simulink model "FDM_Degradation_nmmap"  (R2020b)
settings: Solver=ode23tb  StartTime=0  StopTime=t_final  MaxStep=0.1  RelTol=1e-3
values from neighbouring files (symbols this model uses):
  initial_50_n = repmat(C_avg_n, 1, 49)    [RUn_Model_FDM.m]
settings Model: Creator=moonjihoon  LastModifiedBy=moonjihoon

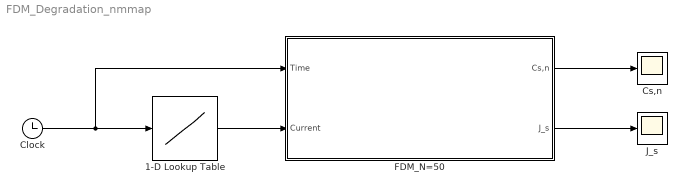
== system FDM_Degradation_nmmap ==
  1-D Lookup Table : Lookup_n-D  NumberOfTableDimensions=1  BreakpointsForDimension1=t  Table=u  InternalRulePriority=Speed  RndMeth=Simplest  InputSameDT=on
  Clock : Clock
  Cs,n : Scope
  FDM_N=50 : Subsystem
  J_s : Scope
  wires:
  1-D Lookup Table/1 -> FDM_N=50/2(Current)
  Clock/1 -> FDM_N=50/1(Time), 1-D Lookup Table/1
  FDM_N=50/2(J_s) -> J_s/1
  FDM_N=50/1(Cs,n) -> Cs,n/1

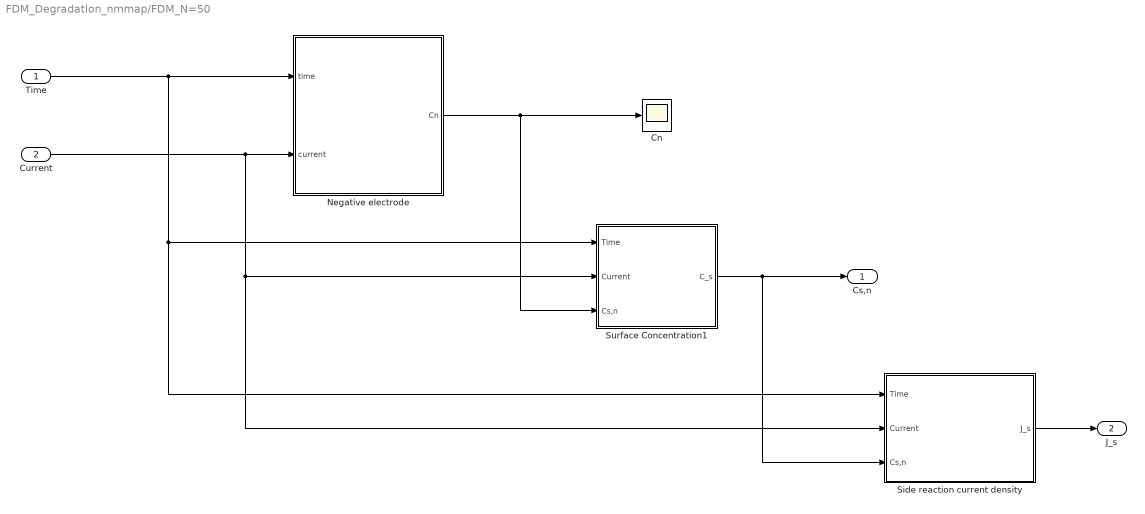
== system FDM_Degradation_nmmap/FDM_N=50 ==
  Time : Inport
  Current : Inport  Port=2
  Cn : Scope
  Negative electrode : Subsystem
  Side reaction current density : Subsystem
  Surface Concentration1 : Subsystem
  Cs,n : Outport
  J_s : Outport  Port=2
  wires:
  Side reaction current density/1(J_s) -> J_s/1
  Surface Concentration1/1(C_s) -> Cs,n/1, Side reaction current density/3(Cs,n)
  Negative electrode/1(Cn) -> Cn/1, Surface Concentration1/3(Cs,n)
  Time/1 -> Surface Concentration1/1(Time), Side reaction current density/1(Time), Negative electrode/1(time)
  Current/1 -> Surface Concentration1/2(Current), Side reaction current density/2(Current), Negative electrode/2(current)

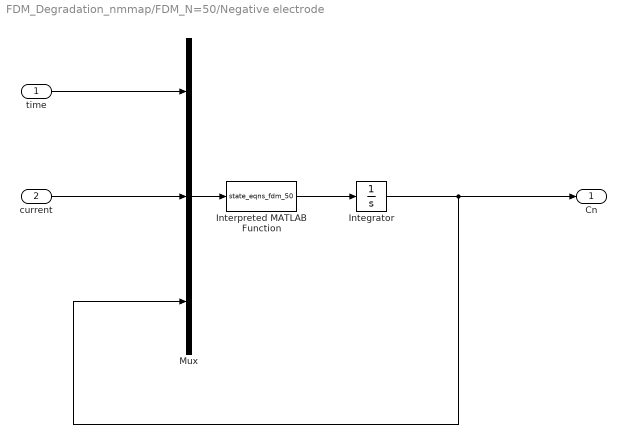
== system FDM_Degradation_nmmap/FDM_N=50/Negative electrode ==
  time : Inport
  current : Inport  Port=2
  Integrator : Integrator  InitialCondition=initial_50_n
  Interpreted MATLAB Function : MATLABFcn  MATLABFcn=state_eqns_fdm_50
  Mux : Mux  Inputs=3
  Cn : Outport
  wires:
  Interpreted MATLAB Function/1 -> Integrator/1
  time/1 -> Mux/1
  current/1 -> Mux/2
  Mux/1 -> Interpreted MATLAB Function/1
  Integrator/1 -> Mux/3, Cn/1

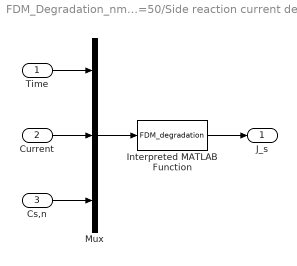
== system FDM_Degradation_nmmap/FDM_N=50/Side reaction current density ==
  Time : Inport
  Current : Inport  Port=2
  Cs,n : Inport  Port=3
  Interpreted MATLAB Function : MATLABFcn  MATLABFcn=FDM_degradation
  Mux : Mux  Inputs=3
  J_s : Outport
  wires:
  Interpreted MATLAB Function/1 -> J_s/1
  Time/1 -> Mux/1
  Current/1 -> Mux/2
  Mux/1 -> Interpreted MATLAB Function/1
  Cs,n/1 -> Mux/3

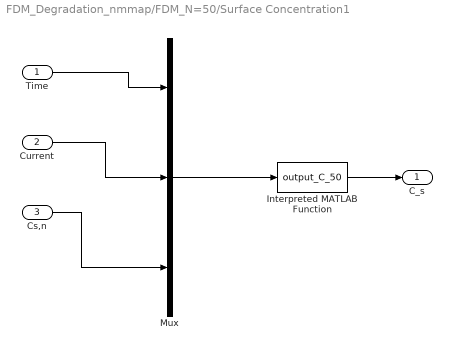
== system FDM_Degradation_nmmap/FDM_N=50/Surface Concentration1 ==
  Time : Inport
  Current : Inport  Port=2
  Cs,n : Inport  Port=3
  Interpreted MATLAB Function : MATLABFcn  MATLABFcn=output_C_50
  Mux : Mux  Inputs=3
  C_s : Outport
  wires:
  Interpreted MATLAB Function/1 -> C_s/1
  Cs,n/1 -> Mux/3
  Current/1 -> Mux/2
  Mux/1 -> Interpreted MATLAB Function/1
  Time/1 -> Mux/1
